simulink model "Validation_Tricopter_Model"  (R2015a)
settings: Solver=ode3  SolverMode=SingleTasking  StartTime=0.0  StopTime=20  FixedStep=T_sim  RelTol=1e-3
PreLoadFcn:
  | LoadLibraries
values from neighbouring files (symbols this model uses):
  a = 10.26    [SetupComplete.m]
  A_x = 0.015    [SetupComplete.m]
  A_y = A_x    (= 0.015)    [SetupComplete.m]
  A_z = 0.16    [SetupComplete.m]
  C_d0 = 0.001193    [SetupComplete.m]
  C_x = 1.2    [SetupComplete.m]
  C_y = C_x    (= 1.2)    [SetupComplete.m]
  C_z = 2.2    [SetupComplete.m]
  CG_0 = [0,0,0.02]'    [SetupComplete.m]
  g = 9.81    [SetupComplete.m]
  h = 0.08    [SetupComplete.m]
  h_FA = 0.02    [SetupComplete.m]
  h_M = 0.064    [SetupComplete.m]
  I_BAC_0 = [ Ix,0,Ixz;0,Iy,0;Ixz,0,Iz]    [SetupComplete.m]
  I_prop = 1/4*M_eq*R^2*diag([1,1,2])    [SetupComplete.m]
  I_tube = [1/2*M_tube*R_tube_eq^2,0,  0  ;           0 ,1/3*M_tube*l_arm^2,0;             0  ,0,1/3*M_tube*l_arm^2]    [SetupComplete.m]
  Initial_Omegas = [1;1;1]*Omega_hover    [Run3Copter.m]
  J_FA = I_prop(1,1) + m_prop*h^2  + m_FA*h_FA^2 + m_M*h_M^2    [SetupComplete.m]
  J_T = J_m+1/2*M_eq*R^2    (= 2.000642e-05)    [SetupComplete.m]
  Ki = lqi(LM_4DOF_aug, Q,R)    [robust_controller.m]
  l = 0.3450    (= 0.345)    [NDI_components.m]    (also in SetupComplete.m; robust_controller.m)
  l_arm = 0.264    [SetupComplete.m]
  m = 3.51    [SetupComplete.m]
  m_0 = 2.61    [SetupComplete.m]
  m_FA = 0.02    [SetupComplete.m]
  m_M = 0.300    (= 0.3)    [SetupComplete.m]
  m_prop = 0.02    [SetupComplete.m]
  R = 0.1778    [SetupComplete.m]    (also in robust_controller.m = eye(4))
  rho = 1.15    [SetupComplete.m]
  sigma = b*c/(pi*R)    (= 0.107416159567)    [SetupComplete.m]
  T_sim = 0.01    [Run3Copter.m]
  theta_0 = 0.38397    [SetupComplete.m]
  theta_1 = -0.2967    [SetupComplete.m]
  trim_simplemodel = [0.589627915568 -2.20656039197 0 0.588313336084 0 0 0.588313330414 0 0]    [trimvalues.mat]
  V_4DOF_last = [0.0122475086001 0.00870447045314 -0.0292257707267 -0.0198753669721 -0.00290766514824 -0.0269511839788 0.0344308792695 -0.0305235710433 -0.0274078219028 -0.0329291952852 -0.0272335702183 -0.00643013158961 ... (1500 elements, 50x30)]    [NN_c_weights.mat]
  v_i0 = sqrt( 1/3*m*g/(2*rho*pi*R^2)  )    [SetupComplete.m]
  W_4DOF_last = [0.0132359246225 -0.0402459595001 -0.0221501781133 0.0046881519205 0.0457506835434 0.0464888535199 -0.0342386918322 0.0470592781761 0.0457166948243 -0.00146243512772 0.0300280468889 -0.0358113661373 ... (204 elements, 4x51)]    [NN_c_weights.mat]
undefined symbols (not defined in the file or in its folder): DOWN_0, EAST_0, Motor, NORTH_0, P_0, Prop, Q_0, R_0, sigmatest, U_0, V_0, v_i_adim, Vx_adim, Vz_adim, W_0
undefined symbols (not defined in the file): Initial_Torques, Rotation_sign, Tau_motors
libraries: simulink x66, XXCopter x32, vrlib x26, simulink_extras x6, Adaptive_FaultTolerantControl x6, qcatlib x4, dspinverses x4, lib_controller x4, aerolib6dofsys x3, aerolibtransform2 x3, aerolib6dof2 x1
(part 9 of 11)

== system Validation_Tricopter_Model/3 Copter Complete/Arms Dynamics: Forces and Moments/4 DOF Arms Dynamics: Forces and Moments1/4 DOF Arms Dynamics: Forces and Moments1/Arm Dynamics2/Aerodynamics Propeller ==
  note: Rotation_sign:
      |
      | * Anticlockwise from above rotation: Rotation_sign= -1
      | * Clockwise from above rotation: Rotation_sign= 1
  Omega : Inport
  h_ground : Inport  Port=2
  r_p : Inport  Port=3
  V^A : Inport  Port=4
  T_FaFb : Inport  Port=5
  2D vec norm : XXCopter/2D vec norm
  2D vec norm1 : XXCopter/2D vec norm
  Abs2 : Abs
  Add : Sum
  Aero Forces and Moments emb : Subsystem  AncestorBlock=XXCopter/Aero Forces and Moments emb  TreatAsAtomicUnit=on
  Dimensionless AB induced Vel Map : Lookup_n-D  BreakpointsForDimension1=Vx_adim  BreakpointsForDimension2=Vz_adim  BreakpointsForDimension3=[5, 7]  Table=v_i_adim  RndMeth=Simplest  InputSameDT=on
  Divide : Product  Inputs=**
  F prop @ Fb : Product  Multiplication=Matrix(*)
  Gain : Gain  Gain=-1
  Gain1 : Gain  Gain=-1
  Induced hover Vel : Constant  Value=v_i0
  M prop @Fb : Product  Multiplication=Matrix(*)
  M_PAF : vrlib/Utilities/Cross Product
  Omega*R : Product  Inputs=**
  Prop Coefficients : MATLAB Function  TreatAsAtomicUnit=on
  Propeller Torque1 : Selector  IndexMode=Zero-based  InputPortWidth=3  Indices=2
  Radius Prop : Constant  Value=R
  Reaction! : Gain  Gain=-1
  Rotation_sign : Constant  Value=Rot_sign
  Sign : Signum
  V_A_x : Selector  InputPortWidth=3  Indices=[1 2]
  V_A_x,y : Selector  InputPortWidth=3  Indices=[1 2]
  V_A_x,y1 : Selector  InputPortWidth=3  Indices=[3]
  V_A_z : Selector  InputPortWidth=3  Indices=3
  Vx dimless : Product  Inputs=*/
  Vz dimless1 : Product  Inputs=*/
  lambda : Sum
  lambdaZ : Product  Inputs=*/
  lambda_i : Product  Inputs=*/
  mu : Product  Inputs=*/
  rho : Constant  Value=rho
  v_i dimension : Product  Inputs=**
  Prop_Torque_out : Outport
  Forces_prop @Fb : Outport  Port=2
  Moments_prop @Fb : Outport  Port=3
  wires:
  Abs2/1 -> Divide/1
  Sign/1 -> Divide/2
  Propeller Torque1/1 -> Abs2/1
  Divide/1 -> Prop_Torque_out/1
  rho/1 -> Aero Forces and Moments emb/7(rho)
  Reaction!/1 -> Aero Forces and Moments emb/9(Moment_sign)
  Prop Coefficients/4(C_Q) -> Aero Forces and Moments emb/4(C_Q), Sign/1
  mu/1 -> Prop Coefficients/2(mu)
  2D vec norm/1 -> Vx dimless/1
  M prop @Fb/1 -> Add/2
  M_PAF/1 -> Add/1
  r_p/1 -> M_PAF/1
  F prop @ Fb/1 -> Forces_prop @Fb/1, M_PAF/2
  Aero Forces and Moments emb/1(Fp) -> F prop @ Fb/2
  T_FaFb/1 -> F prop @ Fb/1, M prop @Fb/1
  Rotation_sign/1 -> Reaction!/1
  h_ground/1 -> Aero Forces and Moments emb/8(h_ground)
  Add/1 -> Moments_prop @Fb/1
  Aero Forces and Moments emb/2("M_PM ") -> Propeller Torque1/1, M prop @Fb/2
  Omega/1 -> Omega*R/2, Aero Forces and Moments emb/5(Omega)
  V^A/1 -> V_A_z/1, V_A_x/1, V_A_x,y1/1, Aero Forces and Moments emb/6(V_A), V_A_x,y/1
  Prop Coefficients/3(C_MH) -> Aero Forces and Moments emb/3(C_MH)
  Prop Coefficients/2(C_H) -> Aero Forces and Moments emb/2(C_H)
  Prop Coefficients/1(C_T) -> Aero Forces and Moments emb/1(C_T)
  lambda/1 -> Prop Coefficients/1(lambda)
  Gain1/1 -> Vz dimless1/1
  lambdaZ/1 -> lambda/2
  lambda_i/1 -> lambda/1
  Gain/1 -> lambdaZ/1
  V_A_x,y1/1 -> Gain/1
  v_i dimension/1 -> lambda_i/1
  Dimensionless AB induced Vel Map/1 -> v_i dimension/1
  Induced hover Vel/1 -> Vx dimless/2, Vz dimless1/2, v_i dimension/2
  V_A_z/1 -> Gain1/1
  Vz dimless1/1 -> Dimensionless AB induced Vel Map/2
  V_A_x/1 -> 2D vec norm/1
  Vx dimless/1 -> Dimensionless AB induced Vel Map/1
  Omega*R/1 -> lambda_i/2, lambdaZ/2, mu/2
  2D vec norm1/1 -> mu/1
  V_A_x,y/1 -> 2D vec norm1/1
  Radius Prop/1 -> Omega*R/1

== system Validation_Tricopter_Model/3 Copter Complete/Arms Dynamics: Forces and Moments/4 DOF Arms Dynamics: Forces and Moments1/4 DOF Arms Dynamics: Forces and Moments1/Arm Dynamics2/Arms Kinematics ==
  Angles (rad) : Inport
  Angles_dot (rad/s) : Inport  Port=2
  Add : Sum
  Add3 : Sum
  Arm_no : Constant  Value=Arm_number
  Cross Product : vrlib/Utilities/Cross Product
  DCM Arm : MATLAB Function  TreatAsAtomicUnit=on
  Demux : Demux  Outputs=2
  Demux3 : Demux  Outputs=2
  Fa->Fb : Product  Multiplication=Matrix(*)
  Gain7 : Gain  Gain=[0;0;-1]
  Hub_position : Constant  Value=Arm_hub_position
  Matrix Multiply : Product  Multiplication=Matrix(*)
  Permute Dimensions : PermuteDimensions
  eta_dir : Gain  Gain=eta_dir
  gamma_dir : Gain  Gain=gamma_dir
  h arm : Constant  Value=h_prop
  r_p (m) : Outport
  r_p_dot (m/s) : Outport  Port=2
  T_F_a,Fb : Outport  Port=3
  omega_Ab (rad/s) : Outport  Port=4
  wires:
  Arm_no/1 -> DCM Arm/1(arm_no)
  Cross Product/1 -> r_p_dot (m/s)/1
  Fa->Fb/1 -> Add3/2, Cross Product/2
  Hub_position/1 -> Add3/1
  Gain7/1 -> Fa->Fb/2
  h arm/1 -> Gain7/1
  Add3/1 -> r_p (m)/1  "r_p (m)"
  Add/1 -> omega_Ab (rad/s)/1, Cross Product/1  "omega_Ab"
  eta_dir/1 -> Add/1
  Matrix Multiply/1 -> Add/2
  gamma_dir/1 -> Matrix Multiply/2
  Demux3/1 -> eta_dir/1  "eta_dot"
  Demux3/2 -> gamma_dir/1  "gamma_dot"
  Angles_dot (rad/s)/1 -> Demux3/1
  Demux/2 -> DCM Arm/3(gamma)
  Demux/1 -> DCM Arm/2(eta)
  Angles (rad)/1 -> Demux/1
  Permute Dimensions/1 -> Fa->Fb/1, Matrix Multiply/1, T_F_a,Fb/1  "T_F_a,Fb"
  DCM Arm/1(T_Fb_FA) -> Permute Dimensions/1

== system Validation_Tricopter_Model/3 Copter Complete/Arms Dynamics: Forces and Moments/4 DOF Arms Dynamics: Forces and Moments1/4 DOF Arms Dynamics: Forces and Moments1/Arm Dynamics2/Servos Dynamics ==
  Com Angles (rad) : Inport
  Torques? : Inport  Port=2
  Add : Sum  Inputs=+-
  Add1 : Sum
  Demux : Demux  Outputs=2
  Derivative{,1..3} (4 alike) : Derivative  CoefficientInTFapproximation=derv_param
  Mux{,1..4} (5 alike) : Mux  Inputs=2
  Terminator : Terminator
  eta_1 : TransferFcn  Numerator=0  Denominator=1
  eta_2 : TransferFcn  Numerator=0  Denominator=1
  init_eta : Constant  Value=init_eta
  init_eta1 : Constant  Value=init_eta
  init_gamma : Constant  Value=init_gamma
  init_gamma1 : Constant  Value=init_gamma
  Angles Arms (rad) : Outport
  Angles_dot (rad/s) : Outport  Port=2
  Angles_dot_dot (rad/s^2) : Outport  Port=3
  wires:
  Com Angles (rad)/1 -> Add/1
  Demux/1 -> eta_1/1
  Demux/2 -> eta_2/1
  eta_1/1 -> Derivative/1, Mux/1
  eta_2/1 -> Mux/2, Derivative1/1
  Mux1/1 -> Angles_dot (rad/s)/1
  Mux2/1 -> Angles_dot_dot (rad/s^2)/1
  Derivative1/1 -> Derivative3/1, Mux1/2
  Derivative2/1 -> Mux2/1
  Derivative3/1 -> Mux2/2
  Derivative/1 -> Mux1/1, Derivative2/1
  Torques?/1 -> Terminator/1
  Add/1 -> Demux/1
  init_eta/1 -> Mux3/1
  Mux3/1 -> Add/2
  init_gamma/1 -> Mux3/2
  init_eta1/1 -> Mux4/1
  init_gamma1/1 -> Mux4/2
  Mux/1 -> Add1/2
  Mux4/1 -> Add1/1
  Add1/1 -> Angles Arms (rad)/1

== system Validation_Tricopter_Model/3 Copter Complete/Arms Dynamics: Forces and Moments/9 DOF Arms Dynamics: Forces and Moments/9 DOF Arms Dynamics: Forces and Moments/Arm Dynamics/Aerodynamics Propeller ==
  note: Rotation_sign:
      |
      | * Anticlockwise from above rotation: Rotation_sign= -1
      | * Clockwise from above rotation: Rotation_sign= 1
  Omega : Inport
  h_ground : Inport  Port=2
  r_p : Inport  Port=3
  V^A : Inport  Port=4
  T_FaFb : Inport  Port=5
  2D vec norm : XXCopter/2D vec norm
  2D vec norm1 : XXCopter/2D vec norm
  Abs2 : Abs
  Add : Sum
  Aero Forces and Moments emb : Subsystem  AncestorBlock=XXCopter/Aero Forces and Moments emb  TreatAsAtomicUnit=on
  Dimensionless AB induced Vel Map : Lookup_n-D  BreakpointsForDimension1=Vx_adim  BreakpointsForDimension2=Vz_adim  BreakpointsForDimension3=[5, 7]  Table=v_i_adim  RndMeth=Simplest  InputSameDT=on
  Divide : Product  Inputs=**
  F prop @ Fb : Product  Multiplication=Matrix(*)
  Gain : Gain  Gain=-1
  Gain1 : Gain  Gain=-1
  Induced hover Vel : Constant  Value=v_i0
  M prop @Fb : Product  Multiplication=Matrix(*)
  M_PAF : vrlib/Utilities/Cross Product
  Omega*R : Product  Inputs=**
  Prop Coefficients : MATLAB Function  TreatAsAtomicUnit=on
  Propeller Torque1 : Selector  IndexMode=Zero-based  InputPortWidth=3  Indices=2
  Radius Prop : Constant  Value=R
  Reaction! : Gain  Gain=-1
  Reaction!1 : Gain  Gain=sigmatest(1,2)
  Reaction!2 : Gain  Gain=sigmatest(1,3)
  Reaction!3 : Gain  Gain=sigmatest(1,4)
  Reaction!4 : Gain  Gain=sigmatest(1,1)
  Rotation_sign : Constant  Value=Rot_sign
  Sign : Signum
  V_A_x : Selector  InputPortWidth=3  Indices=[1 2]
  V_A_x,y : Selector  InputPortWidth=3  Indices=[1 2]
  V_A_x,y1 : Selector  InputPortWidth=3  Indices=[3]
  V_A_z : Selector  InputPortWidth=3  Indices=3
  Vx dimless : Product  Inputs=*/
  Vz dimless1 : Product  Inputs=*/
  lambda : Sum
  lambdaZ : Product  Inputs=*/
  lambda_i : Product  Inputs=*/
  mu : Product  Inputs=*/
  rho : Constant  Value=rho
  v_i dimension : Product  Inputs=**
  Prop_Torque_out : Outport
  Forces_prop @Fb : Outport  Port=2
  Moments_prop @Fb : Outport  Port=3
  wires:
  Abs2/1 -> Divide/1
  Sign/1 -> Divide/2
  Propeller Torque1/1 -> Abs2/1
  Divide/1 -> Prop_Torque_out/1
  rho/1 -> Aero Forces and Moments emb/7(rho)
  Reaction!/1 -> Aero Forces and Moments emb/9(Moment_sign)
  mu/1 -> Prop Coefficients/2(mu)
  2D vec norm/1 -> Vx dimless/1
  M prop @Fb/1 -> Add/2
  M_PAF/1 -> Add/1
  r_p/1 -> M_PAF/1
  F prop @ Fb/1 -> Forces_prop @Fb/1, M_PAF/2
  Aero Forces and Moments emb/1(Fp) -> F prop @ Fb/2
  T_FaFb/1 -> F prop @ Fb/1, M prop @Fb/1
  Rotation_sign/1 -> Reaction!/1
  h_ground/1 -> Aero Forces and Moments emb/8(h_ground)
  Add/1 -> Moments_prop @Fb/1
  Aero Forces and Moments emb/2("M_PM ") -> Propeller Torque1/1, M prop @Fb/2
  Omega/1 -> Omega*R/2, Aero Forces and Moments emb/5(Omega)
  V^A/1 -> V_A_z/1, V_A_x/1, V_A_x,y1/1, Aero Forces and Moments emb/6(V_A), V_A_x,y/1
  lambda/1 -> Prop Coefficients/1(lambda)
  Gain1/1 -> Vz dimless1/1
  lambdaZ/1 -> lambda/2
  lambda_i/1 -> lambda/1
  Gain/1 -> lambdaZ/1
  V_A_x,y1/1 -> Gain/1
  v_i dimension/1 -> lambda_i/1
  Dimensionless AB induced Vel Map/1 -> v_i dimension/1
  Induced hover Vel/1 -> Vx dimless/2, Vz dimless1/2, v_i dimension/2
  V_A_z/1 -> Gain1/1
  Vz dimless1/1 -> Dimensionless AB induced Vel Map/2
  V_A_x/1 -> 2D vec norm/1
  Vx dimless/1 -> Dimensionless AB induced Vel Map/1
  Omega*R/1 -> lambda_i/2, lambdaZ/2, mu/2
  2D vec norm1/1 -> mu/1
  V_A_x,y/1 -> 2D vec norm1/1
  Radius Prop/1 -> Omega*R/1
  Prop Coefficients/1(C_T) -> Reaction!4/1
  Prop Coefficients/2(C_H) -> Reaction!1/1
  Prop Coefficients/3(C_MH) -> Reaction!2/1
  Prop Coefficients/4(C_Q) -> Reaction!3/1
  Reaction!4/1 -> Aero Forces and Moments emb/1(C_T)
  Reaction!1/1 -> Aero Forces and Moments emb/2(C_H)
  Reaction!2/1 -> Aero Forces and Moments emb/3(C_MH)
  Reaction!3/1 -> Aero Forces and Moments emb/4(C_Q), Sign/1

== system Validation_Tricopter_Model/3 Copter Complete/Arms Dynamics: Forces and Moments/9 DOF Arms Dynamics: Forces and Moments/9 DOF Arms Dynamics: Forces and Moments/Arm Dynamics/Arms Kinematics ==
  Angles (rad) : Inport
  Angles_dot (rad/s) : Inport  Port=2
  Add : Sum
  Add3 : Sum
  Arm_no : Constant  Value=Arm_number
  Cross Product : vrlib/Utilities/Cross Product
  DCM Arm : MATLAB Function  TreatAsAtomicUnit=on
  Demux : Demux  Outputs=2
  Demux3 : Demux  Outputs=2
  Fa->Fb : Product  Multiplication=Matrix(*)
  Gain7 : Gain  Gain=[0;0;-1]
  Hub_position : Constant  Value=Arm_hub_position
  Matrix Multiply : Product  Multiplication=Matrix(*)
  Permute Dimensions : PermuteDimensions
  eta_dir : Gain  Gain=eta_dir
  gamma_dir : Gain  Gain=gamma_dir
  h arm : Constant  Value=h_prop
  r_p (m) : Outport
  r_p_dot (m/s) : Outport  Port=2
  T_F_a,Fb : Outport  Port=3
  omega_Ab (rad/s) : Outport  Port=4
  wires:
  Arm_no/1 -> DCM Arm/1(arm_no)
  Cross Product/1 -> r_p_dot (m/s)/1
  Fa->Fb/1 -> Add3/2, Cross Product/2
  Hub_position/1 -> Add3/1
  Gain7/1 -> Fa->Fb/2
  h arm/1 -> Gain7/1
  Add3/1 -> r_p (m)/1  "r_p (m)"
  Add/1 -> omega_Ab (rad/s)/1, Cross Product/1  "omega_Ab"
  eta_dir/1 -> Add/1
  Matrix Multiply/1 -> Add/2
  gamma_dir/1 -> Matrix Multiply/2
  Demux3/1 -> eta_dir/1  "eta_dot"
  Demux3/2 -> gamma_dir/1  "gamma_dot"
  Angles_dot (rad/s)/1 -> Demux3/1
  Demux/2 -> DCM Arm/3(gamma)
  Demux/1 -> DCM Arm/2(eta)
  Angles (rad)/1 -> Demux/1
  Permute Dimensions/1 -> Fa->Fb/1, Matrix Multiply/1, T_F_a,Fb/1  "T_F_a,Fb"
  DCM Arm/1(T_Fb_FA) -> Permute Dimensions/1

== system Validation_Tricopter_Model/3 Copter Complete/Arms Dynamics: Forces and Moments/9 DOF Arms Dynamics: Forces and Moments/9 DOF Arms Dynamics: Forces and Moments/Arm Dynamics/Gyroscopic Moments ==
  T_FAFb : Inport
  omega_A  (rad/s) : Inport  Port=2
  omega_b  (rad/s) : Inport  Port=3
  Angles_dot (rad/s) : Inport  Port=4
  Angles_dot _dot(rad/s^2) : Inport  Port=5
  Omega (rad/s) : Inport  Port=6
  Omega_dot (rad/s^2) : Inport  Port=7
  Arm Inertia1 : MATLAB Function  TreatAsAtomicUnit=on
  Constant : Constant  Value=[l_arm;0;0]
  Cross Product : vrlib/Utilities/Cross Product
  Cross Product1 : vrlib/Utilities/Cross Product
  Demux : Demux  Outputs=2
  Demux1 : Demux  Outputs=2
  Display : Display
  Divide : Product  Inputs=**
  Divide1 : Product  Inputs=**
  F_A->F_b : Product  Multiplication=Matrix(*)
  F_A->F_b1 : Product  Multiplication=Matrix(*)
  Forearm Inertia : Constant  Value=J_FA
  Forearm Inertia1 : Constant  Value=J_FA
  Gain1 : Gain  Gain=[0;0;1]
  Gain3 : Gain  Gain=[0;0;1]
  L_FA : Product  Inputs=**
  L_eta_dot : Product  Multiplication=Matrix(*)
  L_prop : Product  Inputs=**
  Propeller and motor inertia : Constant  Value=J_T
  Propeller and motor inertia1 : Constant  Value=J_T
  "Props, Motor and Forearm L @ F_A" : Sum
  "Props, Motor and Forearm dL/dt @ F_A" : Sum
  Rotation_sign : Constant  Value=Rot_sign
  Rotation_sign1 : Constant  Value=Rot_sign
  Sing of Gyro Moments : Gain  Gain=-1
  Total - Gyro Moment : Sum  Inputs=++++
  d L_FA/dt : Product  Inputs=**
  dL/dt of eta_dot_dot : Product  Multiplication=Matrix(*)
  dL/dt of prop : Product  Inputs=**
  eta_dir : Gain  Gain=eta_dir
  eta_dir1 : Gain  Gain=eta_dir
  gamma_dir : Gain  Gain=gamma_dir
  gamma_dir1 : Gain  Gain=gamma_dir
  M_gyro @Fb : Outport
  wires:
  Angles_dot (rad/s)/1 -> Demux/1
  Angles_dot _dot(rad/s^2)/1 -> Demux1/1
  Demux1/1 -> eta_dir/1  "eta_dot_dot_1"
  Arm Inertia1/1(J_Arm) -> Display/1, dL/dt of eta_dot_dot/1, L_eta_dot/1
  eta_dir/1 -> dL/dt of eta_dot_dot/2
  eta_dir1/1 -> L_eta_dot/2
  Demux/1 -> eta_dir1/1  "eta_dot_1"
  L_eta_dot/1 -> Cross Product/2
  omega_b  (rad/s)/1 -> Cross Product/1
  Demux1/2 -> gamma_dir/1  "gamma_dot_dot_1"
  gamma_dir/1 -> d L_FA/dt/1
  Forearm Inertia/1 -> d L_FA/dt/2
  Omega_dot (rad/s^2)/1 -> Gain3/1  "Omega_dot"
  Divide/1 -> dL/dt of prop/1
  Propeller and motor inertia/1 -> dL/dt of prop/2
  d L_FA/dt/1 -> "Props, Motor and Forearm dL/dt @ F_A"/1
  dL/dt of prop/1 -> "Props, Motor and Forearm dL/dt @ F_A"/2
  Demux/2 -> gamma_dir1/1  "gamma_dot"
  gamma_dir1/1 -> L_FA/1
  Forearm Inertia1/1 -> L_FA/2
  Divide1/1 -> L_prop/1
  Propeller and motor inertia1/1 -> L_prop/2
  L_FA/1 -> "Props, Motor and Forearm L @ F_A"/1
  L_prop/1 -> "Props, Motor and Forearm L @ F_A"/2
  Omega (rad/s)/1 -> Gain1/1  "Omega"
  "Props, Motor and Forearm dL/dt @ F_A"/1 -> F_A->F_b/2
  F_A->F_b/1 -> Total - Gyro Moment/2
  dL/dt of eta_dot_dot/1 -> Total - Gyro Moment/1
  Cross Product/1 -> Total - Gyro Moment/3
  "Props, Motor and Forearm L @ F_A"/1 -> F_A->F_b1/2
  T_FAFb/1 -> Arm Inertia1/1(T_FAFb), F_A->F_b/1, F_A->F_b1/1
  F_A->F_b1/1 -> Cross Product1/2
  omega_A  (rad/s)/1 -> Cross Product1/1
  Cross Product1/1 -> Total - Gyro Moment/4
  Total - Gyro Moment/1 -> Sing of Gyro Moments/1
  Sing of Gyro Moments/1 -> M_gyro @Fb/1
  Constant/1 -> Arm Inertia1/2(Arm_axis)
  Rotation_sign/1 -> Divide/1
  Gain3/1 -> Divide/2
  Rotation_sign1/1 -> Divide1/1
  Gain1/1 -> Divide1/2

== system Validation_Tricopter_Model/3 Copter Complete/Arms Dynamics: Forces and Moments/9 DOF Arms Dynamics: Forces and Moments/9 DOF Arms Dynamics: Forces and Moments/Arm Dynamics1/Aerodynamics Propeller ==
  note: Rotation_sign:
      |
      | * Anticlockwise from above rotation: Rotation_sign= -1
      | * Clockwise from above rotation: Rotation_sign= 1
  Omega : Inport
  h_ground : Inport  Port=2
  r_p : Inport  Port=3
  V^A : Inport  Port=4
  T_FaFb : Inport  Port=5
  2D vec norm : XXCopter/2D vec norm
  2D vec norm1 : XXCopter/2D vec norm
  Abs2 : Abs
  Add : Sum
  Aero Forces and Moments emb : Subsystem  AncestorBlock=XXCopter/Aero Forces and Moments emb  TreatAsAtomicUnit=on
  Dimensionless AB induced Vel Map : Lookup_n-D  BreakpointsForDimension1=Vx_adim  BreakpointsForDimension2=Vz_adim  BreakpointsForDimension3=[5, 7]  Table=v_i_adim  RndMeth=Simplest  InputSameDT=on
  Divide : Product  Inputs=**
  F prop @ Fb : Product  Multiplication=Matrix(*)
  Gain : Gain  Gain=-1
  Gain1 : Gain  Gain=-1
  Induced hover Vel : Constant  Value=v_i0
  M prop @Fb : Product  Multiplication=Matrix(*)
  M_PAF : vrlib/Utilities/Cross Product
  Omega*R : Product  Inputs=**
  Prop Coefficients : MATLAB Function  TreatAsAtomicUnit=on
  Propeller Torque1 : Selector  IndexMode=Zero-based  InputPortWidth=3  Indices=2
  Radius Prop : Constant  Value=R
  Reaction! : Gain  Gain=-1
  Reaction!1 : Gain  Gain=sigmatest(3,1)
  Reaction!2 : Gain  Gain=sigmatest(3,2)
  Reaction!3 : Gain  Gain=sigmatest(3,3)
  Reaction!4 : Gain  Gain=sigmatest(3,4)
  Rotation_sign : Constant  Value=Rot_sign
  Sign : Signum
  V_A_x : Selector  InputPortWidth=3  Indices=[1 2]
  V_A_x,y : Selector  InputPortWidth=3  Indices=[1 2]
  V_A_x,y1 : Selector  InputPortWidth=3  Indices=[3]
  V_A_z : Selector  InputPortWidth=3  Indices=3
  Vx dimless : Product  Inputs=*/
  Vz dimless1 : Product  Inputs=*/
  lambda : Sum
  lambdaZ : Product  Inputs=*/
  lambda_i : Product  Inputs=*/
  mu : Product  Inputs=*/
  rho : Constant  Value=rho
  v_i dimension : Product  Inputs=**
  Prop_Torque_out : Outport
  Forces_prop @Fb : Outport  Port=2
  Moments_prop @Fb : Outport  Port=3
  wires:
  Abs2/1 -> Divide/1
  Sign/1 -> Divide/2
  Propeller Torque1/1 -> Abs2/1
  Divide/1 -> Prop_Torque_out/1
  rho/1 -> Aero Forces and Moments emb/7(rho)
  Reaction!/1 -> Aero Forces and Moments emb/9(Moment_sign)
  Prop Coefficients/4(C_Q) -> Reaction!4/1
  mu/1 -> Prop Coefficients/2(mu)
  2D vec norm/1 -> Vx dimless/1
  M prop @Fb/1 -> Add/2
  M_PAF/1 -> Add/1
  r_p/1 -> M_PAF/1
  F prop @ Fb/1 -> Forces_prop @Fb/1, M_PAF/2
  Aero Forces and Moments emb/1(Fp) -> F prop @ Fb/2
  T_FaFb/1 -> F prop @ Fb/1, M prop @Fb/1
  Rotation_sign/1 -> Reaction!/1
  h_ground/1 -> Aero Forces and Moments emb/8(h_ground)
  Add/1 -> Moments_prop @Fb/1
  Aero Forces and Moments emb/2("M_PM ") -> Propeller Torque1/1, M prop @Fb/2
  Omega/1 -> Omega*R/2, Aero Forces and Moments emb/5(Omega)
  V^A/1 -> V_A_z/1, V_A_x/1, V_A_x,y1/1, Aero Forces and Moments emb/6(V_A), V_A_x,y/1
  Prop Coefficients/3(C_MH) -> Reaction!3/1
  Prop Coefficients/2(C_H) -> Reaction!2/1
  Prop Coefficients/1(C_T) -> Reaction!1/1
  lambda/1 -> Prop Coefficients/1(lambda)
  Gain1/1 -> Vz dimless1/1
  lambdaZ/1 -> lambda/2
  lambda_i/1 -> lambda/1
  Gain/1 -> lambdaZ/1
  V_A_x,y1/1 -> Gain/1
  v_i dimension/1 -> lambda_i/1
  Dimensionless AB induced Vel Map/1 -> v_i dimension/1
  Induced hover Vel/1 -> Vx dimless/2, Vz dimless1/2, v_i dimension/2
  V_A_z/1 -> Gain1/1
  Vz dimless1/1 -> Dimensionless AB induced Vel Map/2
  V_A_x/1 -> 2D vec norm/1
  Vx dimless/1 -> Dimensionless AB induced Vel Map/1
  Omega*R/1 -> lambda_i/2, lambdaZ/2, mu/2
  2D vec norm1/1 -> mu/1
  V_A_x,y/1 -> 2D vec norm1/1
  Radius Prop/1 -> Omega*R/1
  Reaction!1/1 -> Aero Forces and Moments emb/1(C_T)
  Reaction!2/1 -> Aero Forces and Moments emb/2(C_H)
  Reaction!3/1 -> Aero Forces and Moments emb/3(C_MH)
  Reaction!4/1 -> Aero Forces and Moments emb/4(C_Q), Sign/1

== system Validation_Tricopter_Model/3 Copter Complete/Arms Dynamics: Forces and Moments/9 DOF Arms Dynamics: Forces and Moments/9 DOF Arms Dynamics: Forces and Moments/Arm Dynamics1/Arms Kinematics ==
  Angles (rad) : Inport
  Angles_dot (rad/s) : Inport  Port=2
  Add : Sum
  Add3 : Sum
  Arm_no : Constant  Value=Arm_number
  Cross Product : vrlib/Utilities/Cross Product
  DCM Arm : MATLAB Function  TreatAsAtomicUnit=on
  Demux : Demux  Outputs=2
  Demux3 : Demux  Outputs=2
  Fa->Fb : Product  Multiplication=Matrix(*)
  Gain7 : Gain  Gain=[0;0;-1]
  Hub_position : Constant  Value=Arm_hub_position
  Matrix Multiply : Product  Multiplication=Matrix(*)
  Permute Dimensions : PermuteDimensions
  eta_dir : Gain  Gain=eta_dir
  gamma_dir : Gain  Gain=gamma_dir
  h arm : Constant  Value=h_prop
  r_p (m) : Outport
  r_p_dot (m/s) : Outport  Port=2
  T_F_a,Fb : Outport  Port=3
  omega_Ab (rad/s) : Outport  Port=4
  wires:
  Arm_no/1 -> DCM Arm/1(arm_no)
  Cross Product/1 -> r_p_dot (m/s)/1
  Fa->Fb/1 -> Add3/2, Cross Product/2
  Hub_position/1 -> Add3/1
  Gain7/1 -> Fa->Fb/2
  h arm/1 -> Gain7/1
  Add3/1 -> r_p (m)/1  "r_p (m)"
  Add/1 -> omega_Ab (rad/s)/1, Cross Product/1  "omega_Ab"
  eta_dir/1 -> Add/1
  Matrix Multiply/1 -> Add/2
  gamma_dir/1 -> Matrix Multiply/2
  Demux3/1 -> eta_dir/1  "eta_dot"
  Demux3/2 -> gamma_dir/1  "gamma_dot"
  Angles_dot (rad/s)/1 -> Demux3/1
  Demux/2 -> DCM Arm/3(gamma)
  Demux/1 -> DCM Arm/2(eta)
  Angles (rad)/1 -> Demux/1
  Permute Dimensions/1 -> Fa->Fb/1, Matrix Multiply/1, T_F_a,Fb/1  "T_F_a,Fb"
  DCM Arm/1(T_Fb_FA) -> Permute Dimensions/1

== system Validation_Tricopter_Model/3 Copter Complete/Arms Dynamics: Forces and Moments/9 DOF Arms Dynamics: Forces and Moments/9 DOF Arms Dynamics: Forces and Moments/Arm Dynamics1/Gyroscopic Moments ==
  T_FAFb : Inport
  omega_A  (rad/s) : Inport  Port=2
  omega_b  (rad/s) : Inport  Port=3
  Angles_dot (rad/s) : Inport  Port=4
  Angles_dot _dot(rad/s^2) : Inport  Port=5
  Omega (rad/s) : Inport  Port=6
  Omega_dot (rad/s^2) : Inport  Port=7
  Arm Inertia1 : MATLAB Function  TreatAsAtomicUnit=on
  Constant : Constant  Value=[0;l_arm;0]
  Cross Product : vrlib/Utilities/Cross Product
  Cross Product1 : vrlib/Utilities/Cross Product
  Demux : Demux  Outputs=2
  Demux1 : Demux  Outputs=2
  Display : Display
  Divide : Product  Inputs=**
  Divide1 : Product  Inputs=**
  F_A->F_b : Product  Multiplication=Matrix(*)
  F_A->F_b1 : Product  Multiplication=Matrix(*)
  Forearm Inertia : Constant  Value=J_FA
  Forearm Inertia1 : Constant  Value=J_FA
  Gain1 : Gain  Gain=[0;0;1]
  Gain3 : Gain  Gain=[0;0;1]
  L_FA : Product  Inputs=**
  L_eta_dot : Product  Multiplication=Matrix(*)
  L_prop : Product  Inputs=**
  Propeller and motor inertia : Constant  Value=J_T
  Propeller and motor inertia1 : Constant  Value=J_T
  "Props, Motor and Forearm L @ F_A" : Sum
  "Props, Motor and Forearm dL/dt @ F_A" : Sum
  Rotation_sign : Constant  Value=Rot_sign
  Rotation_sign1 : Constant  Value=Rot_sign
  Sing of Gyro Moments : Gain  Gain=-1
  Total - Gyro Moment : Sum  Inputs=++++
  d L_FA/dt : Product  Inputs=**
  dL/dt of eta_dot_dot : Product  Multiplication=Matrix(*)
  dL/dt of prop : Product  Inputs=**
  eta_dir : Gain  Gain=eta_dir
  eta_dir1 : Gain  Gain=eta_dir
  gamma_dir : Gain  Gain=gamma_dir
  gamma_dir1 : Gain  Gain=gamma_dir
  M_gyro @Fb : Outport
  wires:
  Angles_dot (rad/s)/1 -> Demux/1
  Angles_dot _dot(rad/s^2)/1 -> Demux1/1
  Demux1/1 -> eta_dir/1  "eta_dot_dot_1"
  Arm Inertia1/1(J_Arm) -> Display/1, dL/dt of eta_dot_dot/1, L_eta_dot/1
  eta_dir/1 -> dL/dt of eta_dot_dot/2
  eta_dir1/1 -> L_eta_dot/2
  Demux/1 -> eta_dir1/1  "eta_dot_1"
  L_eta_dot/1 -> Cross Product/2
  omega_b  (rad/s)/1 -> Cross Product/1
  Demux1/2 -> gamma_dir/1  "gamma_dot_dot_1"
  gamma_dir/1 -> d L_FA/dt/1
  Forearm Inertia/1 -> d L_FA/dt/2
  Omega_dot (rad/s^2)/1 -> Gain3/1  "Omega_dot"
  Divide/1 -> dL/dt of prop/1
  Propeller and motor inertia/1 -> dL/dt of prop/2
  d L_FA/dt/1 -> "Props, Motor and Forearm dL/dt @ F_A"/1
  dL/dt of prop/1 -> "Props, Motor and Forearm dL/dt @ F_A"/2
  Demux/2 -> gamma_dir1/1  "gamma_dot"
  gamma_dir1/1 -> L_FA/1
  Forearm Inertia1/1 -> L_FA/2
  Divide1/1 -> L_prop/1
  Propeller and motor inertia1/1 -> L_prop/2
  L_FA/1 -> "Props, Motor and Forearm L @ F_A"/1
  L_prop/1 -> "Props, Motor and Forearm L @ F_A"/2
  Omega (rad/s)/1 -> Gain1/1  "Omega"
  "Props, Motor and Forearm dL/dt @ F_A"/1 -> F_A->F_b/2
  F_A->F_b/1 -> Total - Gyro Moment/2
  dL/dt of eta_dot_dot/1 -> Total - Gyro Moment/1
  Cross Product/1 -> Total - Gyro Moment/3
  "Props, Motor and Forearm L @ F_A"/1 -> F_A->F_b1/2
  T_FAFb/1 -> Arm Inertia1/1(T_FAFb), F_A->F_b/1, F_A->F_b1/1
  F_A->F_b1/1 -> Cross Product1/2
  omega_A  (rad/s)/1 -> Cross Product1/1
  Cross Product1/1 -> Total - Gyro Moment/4
  Total - Gyro Moment/1 -> Sing of Gyro Moments/1
  Sing of Gyro Moments/1 -> M_gyro @Fb/1
  Constant/1 -> Arm Inertia1/2(Arm_axis)
  Rotation_sign/1 -> Divide/1
  Gain3/1 -> Divide/2
  Rotation_sign1/1 -> Divide1/1
  Gain1/1 -> Divide1/2

== system Validation_Tricopter_Model/3 Copter Complete/Arms Dynamics: Forces and Moments/9 DOF Arms Dynamics: Forces and Moments/9 DOF Arms Dynamics: Forces and Moments/Arm Dynamics2/Aerodynamics Propeller ==
  note: Rotation_sign:
      |
      | * Anticlockwise from above rotation: Rotation_sign= -1
      | * Clockwise from above rotation: Rotation_sign= 1
  Omega : Inport
  h_ground : Inport  Port=2
  r_p : Inport  Port=3
  V^A : Inport  Port=4
  T_FaFb : Inport  Port=5
  2D vec norm : XXCopter/2D vec norm
  2D vec norm1 : XXCopter/2D vec norm
  Abs2 : Abs
  Add : Sum
  Aero Forces and Moments emb : Subsystem  AncestorBlock=XXCopter/Aero Forces and Moments emb  TreatAsAtomicUnit=on
  Dimensionless AB induced Vel Map : Lookup_n-D  BreakpointsForDimension1=Vx_adim  BreakpointsForDimension2=Vz_adim  BreakpointsForDimension3=[5, 7]  Table=v_i_adim  RndMeth=Simplest  InputSameDT=on
  Divide : Product  Inputs=**
  F prop @ Fb : Product  Multiplication=Matrix(*)
  Gain : Gain  Gain=-1
  Gain1 : Gain  Gain=-1
  Induced hover Vel : Constant  Value=v_i0
  M prop @Fb : Product  Multiplication=Matrix(*)
  M_PAF : vrlib/Utilities/Cross Product
  Omega*R : Product  Inputs=**
  Prop Coefficients : MATLAB Function  TreatAsAtomicUnit=on
  Propeller Torque1 : Selector  IndexMode=Zero-based  InputPortWidth=3  Indices=2
  Radius Prop : Constant  Value=R
  Reaction! : Gain  Gain=-1
  Reaction!1 : Gain  Gain=sigmatest(2,1)
  Reaction!2 : Gain  Gain=sigmatest(2,2)
  Reaction!3 : Gain  Gain=sigmatest(2,3)
  Reaction!4 : Gain  Gain=sigmatest(2,4)
  Rotation_sign : Constant  Value=Rot_sign
  Sign : Signum
  V_A_x : Selector  InputPortWidth=3  Indices=[1 2]
  V_A_x,y : Selector  InputPortWidth=3  Indices=[1 2]
  V_A_x,y1 : Selector  InputPortWidth=3  Indices=[3]
  V_A_z : Selector  InputPortWidth=3  Indices=3
  Vx dimless : Product  Inputs=*/
  Vz dimless1 : Product  Inputs=*/
  lambda : Sum
  lambdaZ : Product  Inputs=*/
  lambda_i : Product  Inputs=*/
  mu : Product  Inputs=*/
  rho : Constant  Value=rho
  v_i dimension : Product  Inputs=**
  Prop_Torque_out : Outport
  Forces_prop @Fb : Outport  Port=2
  Moments_prop @Fb : Outport  Port=3
  wires:
  Abs2/1 -> Divide/1
  Sign/1 -> Divide/2
  Propeller Torque1/1 -> Abs2/1
  Divide/1 -> Prop_Torque_out/1
  rho/1 -> Aero Forces and Moments emb/7(rho)
  Reaction!/1 -> Aero Forces and Moments emb/9(Moment_sign)
  Prop Coefficients/4(C_Q) -> Reaction!4/1
  mu/1 -> Prop Coefficients/2(mu)
  2D vec norm/1 -> Vx dimless/1
  M prop @Fb/1 -> Add/2
  M_PAF/1 -> Add/1
  r_p/1 -> M_PAF/1
  F prop @ Fb/1 -> Forces_prop @Fb/1, M_PAF/2
  Aero Forces and Moments emb/1(Fp) -> F prop @ Fb/2
  T_FaFb/1 -> F prop @ Fb/1, M prop @Fb/1
  Rotation_sign/1 -> Reaction!/1
  h_ground/1 -> Aero Forces and Moments emb/8(h_ground)
  Add/1 -> Moments_prop @Fb/1
  Aero Forces and Moments emb/2("M_PM ") -> Propeller Torque1/1, M prop @Fb/2
  Omega/1 -> Omega*R/2, Aero Forces and Moments emb/5(Omega)
  V^A/1 -> V_A_z/1, V_A_x/1, V_A_x,y1/1, Aero Forces and Moments emb/6(V_A), V_A_x,y/1
  Prop Coefficients/3(C_MH) -> Reaction!3/1
  Prop Coefficients/2(C_H) -> Reaction!2/1
  Prop Coefficients/1(C_T) -> Reaction!1/1
  lambda/1 -> Prop Coefficients/1(lambda)
  Gain1/1 -> Vz dimless1/1
  lambdaZ/1 -> lambda/2
  lambda_i/1 -> lambda/1
  Gain/1 -> lambdaZ/1
  V_A_x,y1/1 -> Gain/1
  v_i dimension/1 -> lambda_i/1
  Dimensionless AB induced Vel Map/1 -> v_i dimension/1
  Induced hover Vel/1 -> Vx dimless/2, Vz dimless1/2, v_i dimension/2
  V_A_z/1 -> Gain1/1
  Vz dimless1/1 -> Dimensionless AB induced Vel Map/2
  V_A_x/1 -> 2D vec norm/1
  Vx dimless/1 -> Dimensionless AB induced Vel Map/1
  Omega*R/1 -> lambda_i/2, lambdaZ/2, mu/2
  2D vec norm1/1 -> mu/1
  V_A_x,y/1 -> 2D vec norm1/1
  Radius Prop/1 -> Omega*R/1
  Reaction!1/1 -> Aero Forces and Moments emb/1(C_T)
  Reaction!3/1 -> Aero Forces and Moments emb/3(C_MH)
  Reaction!2/1 -> Aero Forces and Moments emb/2(C_H)
  Reaction!4/1 -> Aero Forces and Moments emb/4(C_Q), Sign/1

== system Validation_Tricopter_Model/3 Copter Complete/Arms Dynamics: Forces and Moments/9 DOF Arms Dynamics: Forces and Moments/9 DOF Arms Dynamics: Forces and Moments/Arm Dynamics2/Arms Kinematics ==
  Angles (rad) : Inport
  Angles_dot (rad/s) : Inport  Port=2
  Add : Sum
  Add3 : Sum
  Arm_no : Constant  Value=Arm_number
  Cross Product : vrlib/Utilities/Cross Product
  DCM Arm : MATLAB Function  TreatAsAtomicUnit=on
  Demux : Demux  Outputs=2
  Demux3 : Demux  Outputs=2
  Fa->Fb : Product  Multiplication=Matrix(*)
  Gain7 : Gain  Gain=[0;0;-1]
  Hub_position : Constant  Value=Arm_hub_position
  Matrix Multiply : Product  Multiplication=Matrix(*)
  Permute Dimensions : PermuteDimensions
  eta_dir : Gain  Gain=eta_dir
  gamma_dir : Gain  Gain=gamma_dir
  h arm : Constant  Value=h_prop
  r_p (m) : Outport
  r_p_dot (m/s) : Outport  Port=2
  T_F_a,Fb : Outport  Port=3
  omega_Ab (rad/s) : Outport  Port=4
  wires:
  Arm_no/1 -> DCM Arm/1(arm_no)
  Cross Product/1 -> r_p_dot (m/s)/1
  Fa->Fb/1 -> Add3/2, Cross Product/2
  Hub_position/1 -> Add3/1
  Gain7/1 -> Fa->Fb/2
  h arm/1 -> Gain7/1
  Add3/1 -> r_p (m)/1  "r_p (m)"
  Add/1 -> omega_Ab (rad/s)/1, Cross Product/1  "omega_Ab"
  eta_dir/1 -> Add/1
  Matrix Multiply/1 -> Add/2
  gamma_dir/1 -> Matrix Multiply/2
  Demux3/1 -> eta_dir/1  "eta_dot"
  Demux3/2 -> gamma_dir/1  "gamma_dot"
  Angles_dot (rad/s)/1 -> Demux3/1
  Demux/2 -> DCM Arm/3(gamma)
  Demux/1 -> DCM Arm/2(eta)
  Angles (rad)/1 -> Demux/1
  Permute Dimensions/1 -> Fa->Fb/1, Matrix Multiply/1, T_F_a,Fb/1  "T_F_a,Fb"
  DCM Arm/1(T_Fb_FA) -> Permute Dimensions/1

== system Validation_Tricopter_Model/3 Copter Complete/Arms Dynamics: Forces and Moments/9 DOF Arms Dynamics: Forces and Moments/9 DOF Arms Dynamics: Forces and Moments/Arm Dynamics2/Gyroscopic Moments ==
  T_FAFb : Inport
  omega_A  (rad/s) : Inport  Port=2
  omega_b  (rad/s) : Inport  Port=3
  Angles_dot (rad/s) : Inport  Port=4
  Angles_dot _dot(rad/s^2) : Inport  Port=5
  Omega (rad/s) : Inport  Port=6
  Omega_dot (rad/s^2) : Inport  Port=7
  Arm Inertia1 : MATLAB Function  TreatAsAtomicUnit=on
  Constant : Constant  Value=[0;-l_arm;0]
  Cross Product : vrlib/Utilities/Cross Product
  Cross Product1 : vrlib/Utilities/Cross Product
  Demux : Demux  Outputs=2
  Demux1 : Demux  Outputs=2
  Display : Display
  Divide : Product  Inputs=**
  Divide1 : Product  Inputs=**
  F_A->F_b : Product  Multiplication=Matrix(*)
  F_A->F_b1 : Product  Multiplication=Matrix(*)
  Forearm Inertia : Constant  Value=J_FA
  Forearm Inertia1 : Constant  Value=J_FA
  Gain1 : Gain  Gain=[0;0;1]
  Gain3 : Gain  Gain=[0;0;1]
  L_FA : Product  Inputs=**
  L_eta_dot : Product  Multiplication=Matrix(*)
  L_prop : Product  Inputs=**
  Propeller and motor inertia : Constant  Value=J_T
  Propeller and motor inertia1 : Constant  Value=J_T
  "Props, Motor and Forearm L @ F_A" : Sum
  "Props, Motor and Forearm dL/dt @ F_A" : Sum
  Rotation_sign : Constant  Value=Rot_sign
  Rotation_sign1 : Constant  Value=Rot_sign
  Sing of Gyro Moments : Gain  Gain=-1
  Total - Gyro Moment : Sum  Inputs=++++
  d L_FA/dt : Product  Inputs=**
  dL/dt of eta_dot_dot : Product  Multiplication=Matrix(*)
  dL/dt of prop : Product  Inputs=**
  eta_dir : Gain  Gain=eta_dir
  eta_dir1 : Gain  Gain=eta_dir
  gamma_dir : Gain  Gain=gamma_dir
  gamma_dir1 : Gain  Gain=gamma_dir
  M_gyro @Fb : Outport
  wires:
  Angles_dot (rad/s)/1 -> Demux/1
  Angles_dot _dot(rad/s^2)/1 -> Demux1/1
  Demux1/1 -> eta_dir/1  "eta_dot_dot_1"
  Arm Inertia1/1(J_Arm) -> Display/1, dL/dt of eta_dot_dot/1, L_eta_dot/1
  eta_dir/1 -> dL/dt of eta_dot_dot/2
  eta_dir1/1 -> L_eta_dot/2
  Demux/1 -> eta_dir1/1  "eta_dot_1"
  L_eta_dot/1 -> Cross Product/2
  omega_b  (rad/s)/1 -> Cross Product/1
  Demux1/2 -> gamma_dir/1  "gamma_dot_dot_1"
  gamma_dir/1 -> d L_FA/dt/1
  Forearm Inertia/1 -> d L_FA/dt/2
  Omega_dot (rad/s^2)/1 -> Gain3/1  "Omega_dot"
  Divide/1 -> dL/dt of prop/1
  Propeller and motor inertia/1 -> dL/dt of prop/2
  d L_FA/dt/1 -> "Props, Motor and Forearm dL/dt @ F_A"/1
  dL/dt of prop/1 -> "Props, Motor and Forearm dL/dt @ F_A"/2
  Demux/2 -> gamma_dir1/1  "gamma_dot"
  gamma_dir1/1 -> L_FA/1
  Forearm Inertia1/1 -> L_FA/2
  Divide1/1 -> L_prop/1
  Propeller and motor inertia1/1 -> L_prop/2
  L_FA/1 -> "Props, Motor and Forearm L @ F_A"/1
  L_prop/1 -> "Props, Motor and Forearm L @ F_A"/2
  Omega (rad/s)/1 -> Gain1/1  "Omega"
  "Props, Motor and Forearm dL/dt @ F_A"/1 -> F_A->F_b/2
  F_A->F_b/1 -> Total - Gyro Moment/2
  dL/dt of eta_dot_dot/1 -> Total - Gyro Moment/1
  Cross Product/1 -> Total - Gyro Moment/3
  "Props, Motor and Forearm L @ F_A"/1 -> F_A->F_b1/2
  T_FAFb/1 -> Arm Inertia1/1(T_FAFb), F_A->F_b/1, F_A->F_b1/1
  F_A->F_b1/1 -> Cross Product1/2
  omega_A  (rad/s)/1 -> Cross Product1/1
  Cross Product1/1 -> Total - Gyro Moment/4
  Total - Gyro Moment/1 -> Sing of Gyro Moments/1
  Sing of Gyro Moments/1 -> M_gyro @Fb/1
  Constant/1 -> Arm Inertia1/2(Arm_axis)
  Rotation_sign/1 -> Divide/1
  Gain3/1 -> Divide/2
  Rotation_sign1/1 -> Divide1/1
  Gain1/1 -> Divide1/2

== system Validation_Tricopter_Model/3 Copter Complete/Arms Dynamics: Forces and Moments/4 DOF Arms Dynamics: Forces and Moments1/4 DOF Arms Dynamics: Forces and Moments1/Arm Dynamics/Aerodynamics Propeller/Aero Forces and Moments emb ==
  C_T : Inport
  C_H : Inport  Port=2
  C_MH : Inport  Port=3
  C_Q : Inport  Port=4
  Omega : Inport  Port=5
  V_A : Inport  Port=6
  rho : Inport  Port=7
  h_ground : Inport  Port=8
  Moment_sign : Inport  Port=9
  Add : Sum  Inputs=+-
  C_H vec : Product  Inputs=**
  C_MH sign : Product  Inputs=**
  C_Q sign : Product  Inputs=**
  C_T Ground : Product  Inputs=**
  Constant : Constant
  Divide : Product  Inputs=**
  F_p : Product  Inputs=**
  Gain : Gain  Gain=16
  Gain1 : Gain  Gain=-1
  Gain3 : Gain  Gain=-1
  M_PM : Product  Inputs=**
  Math Function : Math  Operator=reciprocal  SaturateOnIntegerOverflow=on
  Math Function1 : Math  Operator=reciprocal  SaturateOnIntegerOverflow=on
  Mh : Product  Inputs=**
  Mux : Mux  Inputs=[2,1]
  Mux1 : Mux  Inputs=[2,1]
  Normalize 2D vector : Subsystem  TreatAsAtomicUnit=on
  R : Constant  Value=R
  V_A_x,y2 : Selector  IndexMode=Zero-based  InputPortWidth=3  Indices=[0,1]
  h^2 : Product  Inputs=**
  omegaR : Product  Inputs=**
  omegaR1 : Product  Inputs=**
  omegaR2 : Product  Inputs=**
  omegaR^2 : Product  Inputs=**
  pi : Constant  Value=pi
  piR^2 : Product  Inputs=**
  rhoS(OmegaR)^2 : Product  Inputs=**
  rhoSR(OmegaR)^2 : Product  Inputs=**
  Fp : Outport
  "M_PM " : Outport  Port=2
  wires:
  R/1 -> rhoSR(OmegaR)^2/2, Divide/2, omegaR/2, Divide/1
  pi/1 -> piR^2/1
  Divide/1 -> omegaR2/2, piR^2/2
  Omega/1 -> omegaR/1
  rho/1 -> omegaR1/1
  omegaR/1 -> omegaR^2/2, omegaR^2/1
  omegaR^2/1 -> omegaR1/2
  piR^2/1 -> rhoS(OmegaR)^2/2
  omegaR1/1 -> rhoS(OmegaR)^2/1
  C_T/1 -> C_T Ground/1
  h_ground/1 -> h^2/2, h^2/1
  h^2/1 -> Gain/1
  Gain/1 -> Math Function/1
  Math Function/1 -> omegaR2/1
  Constant/1 -> Add/1
  omegaR2/1 -> Add/2
  Add/1 -> Math Function1/1
  Math Function1/1 -> C_T Ground/2
  C_T Ground/1 -> Gain1/1
  V_A_x,y2/1 -> Normalize 2D vector/1(v)
  V_A/1 -> V_A_x,y2/1
  Normalize 2D vector/1(normal(v)) -> Gain3/1
  Gain3/1 -> Mh/1, C_H vec/2
  C_H/1 -> C_H vec/1
  C_H vec/1 -> Mux/1
  Gain1/1 -> Mux/2
  Mux/1 -> F_p/1
  rhoS(OmegaR)^2/1 -> rhoSR(OmegaR)^2/1, F_p/2
  C_MH/1 -> C_MH sign/1
  Moment_sign/1 -> C_MH sign/2, C_Q sign/1
  C_MH sign/1 -> Mh/2
  Mh/1 -> Mux1/1
  F_p/1 -> Fp/1
  Mux1/1 -> M_PM/1
  C_Q/1 -> C_Q sign/2
  C_Q sign/1 -> Mux1/2
  rhoSR(OmegaR)^2/1 -> M_PM/2
  M_PM/1 -> "M_PM "/1

== system Validation_Tricopter_Model/3 Copter Complete/Arms Dynamics: Forces and Moments/4 DOF Arms Dynamics: Forces and Moments1/4 DOF Arms Dynamics: Forces and Moments1/Arm Dynamics1/Aerodynamics Propeller/Aero Forces and Moments emb ==
  C_T : Inport
  C_H : Inport  Port=2
  C_MH : Inport  Port=3
  C_Q : Inport  Port=4
  Omega : Inport  Port=5
  V_A : Inport  Port=6
  rho : Inport  Port=7
  h_ground : Inport  Port=8
  Moment_sign : Inport  Port=9
  Add : Sum  Inputs=+-
  C_H vec : Product  Inputs=**
  C_MH sign : Product  Inputs=**
  C_Q sign : Product  Inputs=**
  C_T Ground : Product  Inputs=**
  Constant : Constant
  Divide : Product  Inputs=**
  F_p : Product  Inputs=**
  Gain : Gain  Gain=16
  Gain1 : Gain  Gain=-1
  Gain3 : Gain  Gain=-1
  M_PM : Product  Inputs=**
  Math Function : Math  Operator=reciprocal  SaturateOnIntegerOverflow=on
  Math Function1 : Math  Operator=reciprocal  SaturateOnIntegerOverflow=on
  Mh : Product  Inputs=**
  Mux : Mux  Inputs=[2,1]
  Mux1 : Mux  Inputs=[2,1]
  Normalize 2D vector : Subsystem  TreatAsAtomicUnit=on
  R : Constant  Value=R
  V_A_x,y2 : Selector  IndexMode=Zero-based  InputPortWidth=3  Indices=[0,1]
  h^2 : Product  Inputs=**
  omegaR : Product  Inputs=**
  omegaR1 : Product  Inputs=**
  omegaR2 : Product  Inputs=**
  omegaR^2 : Product  Inputs=**
  pi : Constant  Value=pi
  piR^2 : Product  Inputs=**
  rhoS(OmegaR)^2 : Product  Inputs=**
  rhoSR(OmegaR)^2 : Product  Inputs=**
  Fp : Outport
  "M_PM " : Outport  Port=2
  wires:
  R/1 -> rhoSR(OmegaR)^2/2, Divide/2, omegaR/2, Divide/1
  pi/1 -> piR^2/1
  Divide/1 -> omegaR2/2, piR^2/2
  Omega/1 -> omegaR/1
  rho/1 -> omegaR1/1
  omegaR/1 -> omegaR^2/2, omegaR^2/1
  omegaR^2/1 -> omegaR1/2
  piR^2/1 -> rhoS(OmegaR)^2/2
  omegaR1/1 -> rhoS(OmegaR)^2/1
  C_T/1 -> C_T Ground/1
  h_ground/1 -> h^2/2, h^2/1
  h^2/1 -> Gain/1
  Gain/1 -> Math Function/1
  Math Function/1 -> omegaR2/1
  Constant/1 -> Add/1
  omegaR2/1 -> Add/2
  Add/1 -> Math Function1/1
  Math Function1/1 -> C_T Ground/2
  C_T Ground/1 -> Gain1/1
  V_A_x,y2/1 -> Normalize 2D vector/1(v)
  V_A/1 -> V_A_x,y2/1
  Normalize 2D vector/1(normal(v)) -> Gain3/1
  Gain3/1 -> Mh/1, C_H vec/2
  C_H/1 -> C_H vec/1
  C_H vec/1 -> Mux/1
  Gain1/1 -> Mux/2
  Mux/1 -> F_p/1
  rhoS(OmegaR)^2/1 -> rhoSR(OmegaR)^2/1, F_p/2
  C_MH/1 -> C_MH sign/1
  Moment_sign/1 -> C_MH sign/2, C_Q sign/1
  C_MH sign/1 -> Mh/2
  Mh/1 -> Mux1/1
  F_p/1 -> Fp/1
  Mux1/1 -> M_PM/1
  C_Q/1 -> C_Q sign/2
  C_Q sign/1 -> Mux1/2
  rhoSR(OmegaR)^2/1 -> M_PM/2
  M_PM/1 -> "M_PM "/1

== system Validation_Tricopter_Model/3 Copter Complete/Arms Dynamics: Forces and Moments/4 DOF Arms Dynamics: Forces and Moments1/4 DOF Arms Dynamics: Forces and Moments1/Arm Dynamics2/Aerodynamics Propeller/Aero Forces and Moments emb ==
  C_T : Inport
  C_H : Inport  Port=2
  C_MH : Inport  Port=3
  C_Q : Inport  Port=4
  Omega : Inport  Port=5
  V_A : Inport  Port=6
  rho : Inport  Port=7
  h_ground : Inport  Port=8
  Moment_sign : Inport  Port=9
  Add : Sum  Inputs=+-
  C_H vec : Product  Inputs=**
  C_MH sign : Product  Inputs=**
  C_Q sign : Product  Inputs=**
  C_T Ground : Product  Inputs=**
  Constant : Constant
  Divide : Product  Inputs=**
  F_p : Product  Inputs=**
  Gain : Gain  Gain=16
  Gain1 : Gain  Gain=-1
  Gain3 : Gain  Gain=-1
  M_PM : Product  Inputs=**
  Math Function : Math  Operator=reciprocal  SaturateOnIntegerOverflow=on
  Math Function1 : Math  Operator=reciprocal  SaturateOnIntegerOverflow=on
  Mh : Product  Inputs=**
  Mux : Mux  Inputs=[2,1]
  Mux1 : Mux  Inputs=[2,1]
  Normalize 2D vector : Subsystem  TreatAsAtomicUnit=on
  R : Constant  Value=R
  V_A_x,y2 : Selector  IndexMode=Zero-based  InputPortWidth=3  Indices=[0,1]
  h^2 : Product  Inputs=**
  omegaR : Product  Inputs=**
  omegaR1 : Product  Inputs=**
  omegaR2 : Product  Inputs=**
  omegaR^2 : Product  Inputs=**
  pi : Constant  Value=pi
  piR^2 : Product  Inputs=**
  rhoS(OmegaR)^2 : Product  Inputs=**
  rhoSR(OmegaR)^2 : Product  Inputs=**
  Fp : Outport
  "M_PM " : Outport  Port=2
  wires:
  R/1 -> rhoSR(OmegaR)^2/2, Divide/2, omegaR/2, Divide/1
  pi/1 -> piR^2/1
  Divide/1 -> omegaR2/2, piR^2/2
  Omega/1 -> omegaR/1
  rho/1 -> omegaR1/1
  omegaR/1 -> omegaR^2/2, omegaR^2/1
  omegaR^2/1 -> omegaR1/2
  piR^2/1 -> rhoS(OmegaR)^2/2
  omegaR1/1 -> rhoS(OmegaR)^2/1
  C_T/1 -> C_T Ground/1
  h_ground/1 -> h^2/2, h^2/1
  h^2/1 -> Gain/1
  Gain/1 -> Math Function/1
  Math Function/1 -> omegaR2/1
  Constant/1 -> Add/1
  omegaR2/1 -> Add/2
  Add/1 -> Math Function1/1
  Math Function1/1 -> C_T Ground/2
  C_T Ground/1 -> Gain1/1
  V_A_x,y2/1 -> Normalize 2D vector/1(v)
  V_A/1 -> V_A_x,y2/1
  Normalize 2D vector/1(normal(v)) -> Gain3/1
  Gain3/1 -> Mh/1, C_H vec/2
  C_H/1 -> C_H vec/1
  C_H vec/1 -> Mux/1
  Gain1/1 -> Mux/2
  Mux/1 -> F_p/1
  rhoS(OmegaR)^2/1 -> rhoSR(OmegaR)^2/1, F_p/2
  C_MH/1 -> C_MH sign/1
  Moment_sign/1 -> C_MH sign/2, C_Q sign/1
  C_MH sign/1 -> Mh/2
  Mh/1 -> Mux1/1
  F_p/1 -> Fp/1
  Mux1/1 -> M_PM/1
  C_Q/1 -> C_Q sign/2
  C_Q sign/1 -> Mux1/2
  rhoSR(OmegaR)^2/1 -> M_PM/2
  M_PM/1 -> "M_PM "/1

== system Validation_Tricopter_Model/3 Copter Complete/Arms Dynamics: Forces and Moments/9 DOF Arms Dynamics: Forces and Moments/9 DOF Arms Dynamics: Forces and Moments/Arm Dynamics/Aerodynamics Propeller/Aero Forces and Moments emb ==
  C_T : Inport
  C_H : Inport  Port=2
  C_MH : Inport  Port=3
  C_Q : Inport  Port=4
  Omega : Inport  Port=5
  V_A : Inport  Port=6
  rho : Inport  Port=7
  h_ground : Inport  Port=8
  Moment_sign : Inport  Port=9
  Add : Sum  Inputs=+-
  C_H vec : Product  Inputs=**
  C_MH sign : Product  Inputs=**
  C_Q sign : Product  Inputs=**
  C_T Ground : Product  Inputs=**
  Constant : Constant
  Divide : Product  Inputs=**
  F_p : Product  Inputs=**
  Gain : Gain  Gain=16
  Gain1 : Gain  Gain=-1
  Gain3 : Gain  Gain=-1
  M_PM : Product  Inputs=**
  Math Function : Math  Operator=reciprocal  SaturateOnIntegerOverflow=on
  Math Function1 : Math  Operator=reciprocal  SaturateOnIntegerOverflow=on
  Mh : Product  Inputs=**
  Mux : Mux  Inputs=[2,1]
  Mux1 : Mux  Inputs=[2,1]
  Normalize 2D vector : Subsystem  TreatAsAtomicUnit=on
  R : Constant  Value=R
  V_A_x,y2 : Selector  IndexMode=Zero-based  InputPortWidth=3  Indices=[0,1]
  h^2 : Product  Inputs=**
  omegaR : Product  Inputs=**
  omegaR1 : Product  Inputs=**
  omegaR2 : Product  Inputs=**
  omegaR^2 : Product  Inputs=**
  pi : Constant  Value=pi
  piR^2 : Product  Inputs=**
  rhoS(OmegaR)^2 : Product  Inputs=**
  rhoSR(OmegaR)^2 : Product  Inputs=**
  Fp : Outport
  "M_PM " : Outport  Port=2
  wires:
  R/1 -> rhoSR(OmegaR)^2/2, Divide/2, omegaR/2, Divide/1
  pi/1 -> piR^2/1
  Divide/1 -> omegaR2/2, piR^2/2
  Omega/1 -> omegaR/1
  rho/1 -> omegaR1/1
  omegaR/1 -> omegaR^2/2, omegaR^2/1
  omegaR^2/1 -> omegaR1/2
  piR^2/1 -> rhoS(OmegaR)^2/2
  omegaR1/1 -> rhoS(OmegaR)^2/1
  C_T/1 -> C_T Ground/1
  h_ground/1 -> h^2/2, h^2/1
  h^2/1 -> Gain/1
  Gain/1 -> Math Function/1
  Math Function/1 -> omegaR2/1
  Constant/1 -> Add/1
  omegaR2/1 -> Add/2
  Add/1 -> Math Function1/1
  Math Function1/1 -> C_T Ground/2
  C_T Ground/1 -> Gain1/1
  V_A_x,y2/1 -> Normalize 2D vector/1(v)
  V_A/1 -> V_A_x,y2/1
  Normalize 2D vector/1(normal(v)) -> Gain3/1
  Gain3/1 -> Mh/1, C_H vec/2
  C_H/1 -> C_H vec/1
  C_H vec/1 -> Mux/1
  Gain1/1 -> Mux/2
  Mux/1 -> F_p/1
  rhoS(OmegaR)^2/1 -> rhoSR(OmegaR)^2/1, F_p/2
  C_MH/1 -> C_MH sign/1
  Moment_sign/1 -> C_MH sign/2, C_Q sign/1
  C_MH sign/1 -> Mh/2
  Mh/1 -> Mux1/1
  F_p/1 -> Fp/1
  Mux1/1 -> M_PM/1
  C_Q/1 -> C_Q sign/2
  C_Q sign/1 -> Mux1/2
  rhoSR(OmegaR)^2/1 -> M_PM/2
  M_PM/1 -> "M_PM "/1

== system Validation_Tricopter_Model/3 Copter Complete/Arms Dynamics: Forces and Moments/9 DOF Arms Dynamics: Forces and Moments/9 DOF Arms Dynamics: Forces and Moments/Arm Dynamics1/Aerodynamics Propeller/Aero Forces and Moments emb ==
  C_T : Inport
  C_H : Inport  Port=2
  C_MH : Inport  Port=3
  C_Q : Inport  Port=4
  Omega : Inport  Port=5
  V_A : Inport  Port=6
  rho : Inport  Port=7
  h_ground : Inport  Port=8
  Moment_sign : Inport  Port=9
  Add : Sum  Inputs=+-
  C_H vec : Product  Inputs=**
  C_MH sign : Product  Inputs=**
  C_Q sign : Product  Inputs=**
  C_T Ground : Product  Inputs=**
  Constant : Constant
  Divide : Product  Inputs=**
  F_p : Product  Inputs=**
  Gain : Gain  Gain=16
  Gain1 : Gain  Gain=-1
  Gain3 : Gain  Gain=-1
  M_PM : Product  Inputs=**
  Math Function : Math  Operator=reciprocal  SaturateOnIntegerOverflow=on
  Math Function1 : Math  Operator=reciprocal  SaturateOnIntegerOverflow=on
  Mh : Product  Inputs=**
  Mux : Mux  Inputs=[2,1]
  Mux1 : Mux  Inputs=[2,1]
  Normalize 2D vector : Subsystem  TreatAsAtomicUnit=on
  R : Constant  Value=R
  V_A_x,y2 : Selector  IndexMode=Zero-based  InputPortWidth=3  Indices=[0,1]
  h^2 : Product  Inputs=**
  omegaR : Product  Inputs=**
  omegaR1 : Product  Inputs=**
  omegaR2 : Product  Inputs=**
  omegaR^2 : Product  Inputs=**
  pi : Constant  Value=pi
  piR^2 : Product  Inputs=**
  rhoS(OmegaR)^2 : Product  Inputs=**
  rhoSR(OmegaR)^2 : Product  Inputs=**
  Fp : Outport
  "M_PM " : Outport  Port=2
  wires:
  R/1 -> rhoSR(OmegaR)^2/2, Divide/2, omegaR/2, Divide/1
  pi/1 -> piR^2/1
  Divide/1 -> omegaR2/2, piR^2/2
  Omega/1 -> omegaR/1
  rho/1 -> omegaR1/1
  omegaR/1 -> omegaR^2/2, omegaR^2/1
  omegaR^2/1 -> omegaR1/2
  piR^2/1 -> rhoS(OmegaR)^2/2
  omegaR1/1 -> rhoS(OmegaR)^2/1
  C_T/1 -> C_T Ground/1
  h_ground/1 -> h^2/2, h^2/1
  h^2/1 -> Gain/1
  Gain/1 -> Math Function/1
  Math Function/1 -> omegaR2/1
  Constant/1 -> Add/1
  omegaR2/1 -> Add/2
  Add/1 -> Math Function1/1
  Math Function1/1 -> C_T Ground/2
  C_T Ground/1 -> Gain1/1
  V_A_x,y2/1 -> Normalize 2D vector/1(v)
  V_A/1 -> V_A_x,y2/1
  Normalize 2D vector/1(normal(v)) -> Gain3/1
  Gain3/1 -> Mh/1, C_H vec/2
  C_H/1 -> C_H vec/1
  C_H vec/1 -> Mux/1
  Gain1/1 -> Mux/2
  Mux/1 -> F_p/1
  rhoS(OmegaR)^2/1 -> rhoSR(OmegaR)^2/1, F_p/2
  C_MH/1 -> C_MH sign/1
  Moment_sign/1 -> C_MH sign/2, C_Q sign/1
  C_MH sign/1 -> Mh/2
  Mh/1 -> Mux1/1
  F_p/1 -> Fp/1
  Mux1/1 -> M_PM/1
  C_Q/1 -> C_Q sign/2
  C_Q sign/1 -> Mux1/2
  rhoSR(OmegaR)^2/1 -> M_PM/2
  M_PM/1 -> "M_PM "/1
